simulink model "rlc_sps_sl"  (R2014a)
settings: Solver=ode23tb  StartTime=0.0  StopTime=1  MaxStep=0.1  RelTol=1e-4
PreLoadFcn:
  | Vs = 30;
  | L = 1e-3;
  | C = 1e-3;
  | R = 1;
  | sys = power_analyze('rlc_sps','structure');
libraries: powerlib x7
settings Model: Creator=gdudgeon  LastModifiedBy=cosorio
settings DataIOCC: SignalLoggingSaveFormat=ModelDataLogs  SaveTime=off
settings OptimizationCC: ExpressionDepthLimit=2147483647
settings DebuggingCC: UnderspecifiedInitializationDetection=Classic  FcnCallInpInsideContextMsg=UseLocalSettings  StateNameClashWarn=warning
settings GRTTargetCC: CombineOutputUpdateFcns=off  GRTInterface=on

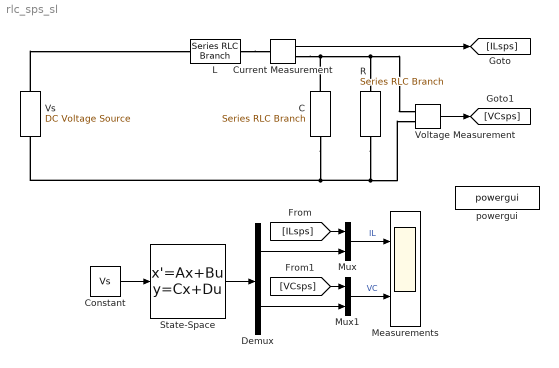
== system rlc_sps_sl ==
  C : powerlib/Elements/Series RLC Branch  LConnTagsString=__new0  RConnTagsString=__new0  BranchType=C  Resistance=R  Inductance=1e-3  SetiL0=off  InitialCurrent=0  Capacitance=C  Setx0=off  InitialVoltage=0  Measurements=None
  Constant : Constant  Value=Vs
  Current Measurement : powerlib/Measurements/Current Measurement  PhasorSimulation=off  OutputType=Complex  PSBequivalent=0
  Demux : Demux  Outputs=2
  L : powerlib/Elements/Series RLC Branch  LConnTagsString=__new0  RConnTagsString=__new0  BranchType=L  Resistance=1  Inductance=L  SetiL0=off  InitialCurrent=0  Capacitance=1e-6  Setx0=off  InitialVoltage=0  Measurements=None
  Measurements : Scope  NumInputPorts=2
      settings: YMin=0~0  YMax=40~40
  Mux : Mux  Inputs=2
  Mux1 : Mux  Inputs=2
  R : powerlib/Elements/Series RLC Branch  LConnTagsString=__new0  RConnTagsString=__new0  BranchType=R  Resistance=R  Inductance=1e-3  SetiL0=off  InitialCurrent=0  Capacitance=1e-6  Setx0=off  InitialVoltage=0  Measurements=None
  State-Space : StateSpace  A=sys.A  B=sys.B  C=sys.C  D=sys.D  X0=sys.x0
  Voltage Measurement : powerlib/Measurements/Voltage Measurement  PhasorSimulation=off  OutputType=Complex  PSBequivalent=0
  Vs : powerlib/Electrical Sources/DC Voltage Source  Amplitude=Vs  Measurements=None
  powergui : powerlib/powergui  SimulationMode=Continuous  SolverType=Tustin  SampleTime=50e-6  frequency=60  SPID=off  DisableSnubberDevices=off  DisableRonSwitches=off  DisableVfSwitches=off  SwTol=0  Interpol=off  DisplayEquations=off  Ts=0  methode=off  frequencyindice=0  Pbase=100e6  ErrMax=1e-4  Iterations=50  UnitsV=kV  UnitsW=MW  FunctionMessages=off  echomessages=off  HookPort=off  EnableUseOfTLC=off  x0status=blocks  RestoreLinks=warning  ResistiveCurrentMeasurement=off  Frange=[0:2:500]  Ylog=off  Xlog=on  ShowGrid=off  save=off  variable=ZData  structure=0  ZoomFFT=on  StartTime=0.0  cycles=1  DisplayStyle=1  fundamental=60  FreqAxis=off  MaxFrequency=1000  frequencyindicesteady=1  RmsSteady=1  display=off
  wires:
  Current Measurement/1 -> [ILsps]
  Voltage Measurement/1 -> [VCsps]
  Constant/1 -> State-Space/1
  State-Space/1 -> Demux/1
  Demux/1 -> Mux/2
  Demux/2 -> Mux1/2
  Mux/1 -> Measurements/1  "IL"
  Mux1/1 -> Measurements/2  "VC"
  [ILsps] -> Mux/1
  [VCsps] -> Mux1/1
  connections:
  Vs/RConn1 -- L/LConn1
  L/RConn1 -- Current Measurement/LConn1
  Current Measurement/RConn1 -- C/LConn1 -- R/LConn1 -- Voltage Measurement/LConn1
  R/RConn1 -- Voltage Measurement/LConn2 -- C/RConn1 -- Vs/LConn1
